simulink model "Wiper_Harness"  (R2022b)
settings: Solver=FixedStepDiscrete  StartTime=0.0  StopTime=10.0  FixedStep=0.1  RelTol=1e-3
settings Model: Creator=suha274823  LastModifiedBy=suha274823
settings OptimizationCC: ReuseModelBlockBuffer=on

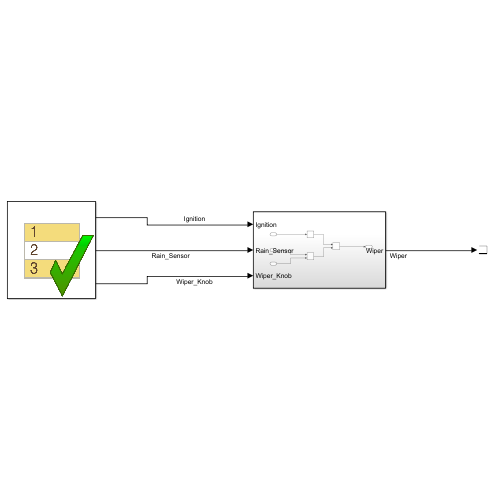
[thumbnail: Simulink's stored preview of the top-level diagram]
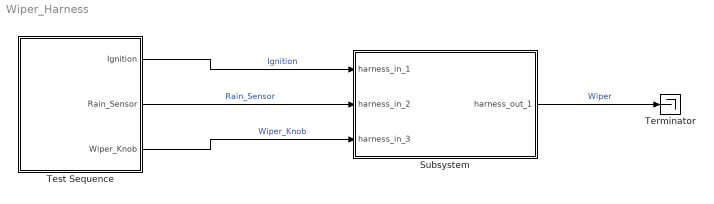
== system Wiper_Harness ==
  Subsystem : Subsystem  Tag=__SL_testing_harness_stub_
  Terminator : Terminator
  Test Sequence : Test Sequence  TreatAsAtomicUnit=on
  wires:
  Test Sequence/1(Ignition) -> Subsystem/1(harness_in_1)  "Ignition"
  Test Sequence/2(Rain_Sensor) -> Subsystem/2(harness_in_2)  "Rain_Sensor"
  Test Sequence/3(Wiper_Knob) -> Subsystem/3(harness_in_3)  "Wiper_Knob"
  Subsystem/1(harness_out_1) -> Terminator/1  "Wiper"

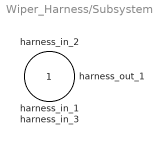
== system Wiper_Harness/Subsystem ==
  harness_in_1 : Inport
  harness_in_2 : Inport  Port=2
  harness_in_3 : Inport  Port=3
  harness_out_1 : Outport

== stateflow chart Wiper_Harness/Test Sequence ==
  settings: updateMethod=DISCRETE  sampleTime=0.1
  state Run
    %% Initialize data outputs.
    Ignition = 0;
    Rain_Sensor = false;
    Wiper_Knob = false;
  state step_1
    Ignition = 1;
    Rain_Sensor = false;
    Wiper_Knob = false;
  state step_2
    Ignition = 1;
    Rain_Sensor = false;
    Wiper_Knob = true;
  state step_3
    Ignition = 1;
    Rain_Sensor = true;
    Wiper_Knob = false;
  state step_4
    Ignition = 1;
    Rain_Sensor = true;
    Wiper_Knob = true;
  (default) -> Run
  (junction 33) -> Run
  (junction 35) -> (junction 33)
  Run -> step_1 : [
      | after(1,sec)
      | ]
  step_1 -> step_2 : [
      | after(1,sec)
      | ]
  step_2 -> step_3 : [
      | after(1,sec)
      | ]
  step_3 -> step_4 : [
      | after(1,sec)
      | ]
  step_4 -> (junction 35) : [
      | after(1,sec)
      | ]
  data: Ignition output double size=[1]; Rain_Sensor output boolean size=[1]; Wiper_Knob output boolean size=[1]
